simulink model "Simul_BASE_XLS_animation"  (R2016b)
settings: Solver=FixedStepAuto  StartTime=0.0  StopTime=60  FixedStep=0.1  RelTol=1e-3  EnableMultiTasking=on
values from neighbouring files (symbols this model uses):
  attitude_0 = [0,0,0]    [ga_detumbling.m]    (also in ga_detumbling_fit.m = [0.0524,-0.0349,0.0175]; ga_pid.m; ga_pid_fit.m; ga_pid_test.m)
  attitude_rate_0 = [0,6.7e-05,0.0041]    [ga_detumbling.m]    (also in ga_detumbling_fit.m = [0.0873,-0.0873,-0.0873]; ga_pid.m; ga_pid_fit.m; ga_pid_test.m)
  dp = x(2)    [ga_detumbling.m]    (also in ga_detumbling_fit.m = d(2); ga_pid.m = x(4); ga_pid_fit.m = d(4); ga_pid_test.m = x(4))
  dr = x(1)    [ga_detumbling.m]    (also in ga_detumbling_fit.m = d(1); ga_pid.m = x(2); ga_pid_fit.m = d(2); ga_pid_test.m = x(2))
  dy = x(3)    [ga_detumbling.m]    (also in ga_detumbling_fit.m = d(3); ga_pid.m = x(6); ga_pid_fit.m = d(6); ga_pid_test.m = x(6))
  override = 2    [ga_pid_fit.m]    (also in ga_pid_test.m; init_var.m)
  pp = x(3)    [ga_pid.m]    (also in ga_pid_fit.m = d(3); ga_pid_test.m; init_var.m = 0.6885)
  pr = x(1)    [ga_pid.m]    (also in ga_pid_fit.m = d(1); ga_pid_test.m; init_var.m = 0.8646)
  py = x(5)    [ga_pid.m]    (also in ga_pid_fit.m = d(5); ga_pid_test.m; init_var.m = 0.371)
  slew = [60 0 0]    [ga_detumbling.m]    (also in ga_pid.m; ga_pid_fit.m; ga_pid_test.m)
libraries: simulink_extras x10, aerolibanim x1, simulink x1, aerolibutil x1
CloseFcn:
  | rtwprivate ssgencode ModelCloseRequest Simul_BASE_3MW
settings Model: Creator=Kendrick  LastModifiedBy=ehernandez
settings SolverCC: MaxConsecutiveMinStep=5  ZeroCrossAlgorithm=Adaptive
settings DataIOCC: LimitDataPoints=on  SaveFormat=Array  SignalLoggingSaveFormat=ModelDataLogs
settings OptimizationCC: ExpressionDepthLimit=2147483647  LifeSpan=inf
settings DebuggingCC: AlgebraicLoopMsg=none  UnderspecifiedInitializationDetection=Classic  MergeDetectMultiDrivingBlocksExec=none  SolverPrmCheckMsg=warning  FcnCallInpInsideContextMsg=warning  StateNameClashWarn=warning  SFUnexpectedBacktrackingDiag=warning  SFNoUnconditionalDefaultTransitionDiag=warning  SFExecutionAtInitializationDiag=none
settings HardwareCC: ProdBitPerInt=16  ProdBitPerPointer=16  ProdBitPerSizeT=16  ProdBitPerPtrDiffT=16  ProdLargestAtomicFloat=None  ProdIntDivRoundTo=Undefined  ProdEndianess=Unspecified  ProdWordSize=16  ProdHWDeviceType=Generic->16-bit Embedded Processor
settings ModelReferenceCC: PropagateSignalLabelsOutOfModel=off
settings GRTTargetCC: TargetLangStandard=C89/C90 (ANSI)  GeneratePreprocessorConditionals=Disable all  CombineOutputUpdateFcns=off  GRTInterface=on
settings ConfigComp: CovMetricSettings=dw  CovHtmlReporting=on  CovSaveCumulativeToWorkspaceVar=on  CovSaveSingleToWorkspaceVar=on  CovExternalEMLEnable=off
settings SimscapeCC: ExplicitSolverDiagnosticOptions=error  GlobalZcOffDiagnosticOptions=error
settings SimMechanicsCC: VisOnUpdateDiagram=on  VisDuringSimulation=on  LastVizWinPosition=[824 49 610 743]  CamPosition=[0.0449883;0.218364;11.4685;]  CamTarget=[-0.000193585;-0.0218554;-0.00055518;]  CamUpVector=[-0.0100593;0.999731;-0.0208998;]  CamHeight=0.706401  VisBackgroundColor=[0.9;0.9;0.95;]  DefaultBodyColor=[1;0;0;]
settings ConfigurationSet: Description=SimMechanics 2G

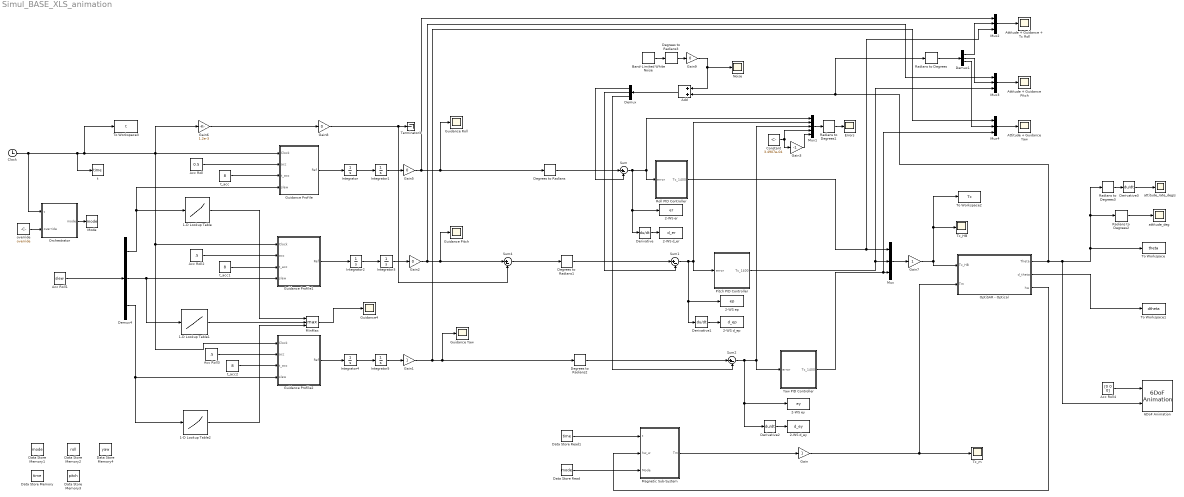
== system Simul_BASE_XLS_animation ==
  1-D Lookup Table : Lookup_n-D  NumberOfTableDimensions=1  BreakpointsForDimension1=[0,10,20,30,60,90]  Table=[0,18,22,25,30,34]  InterpMethod=Cubic spline  ExtrapMethod=Cubic spline  InternalRulePriority=Speed  RndMeth=Simplest  InputSameDT=on
  1-D Lookup Table1 : Lookup_n-D  NumberOfTableDimensions=1  BreakpointsForDimension1=[0,30,60,90]  Table=[0,25,30,34]  InterpMethod=Cubic spline  ExtrapMethod=Cubic spline  InternalRulePriority=Speed  RndMeth=Simplest  InputSameDT=on
  1-D Lookup Table2 : Lookup_n-D  NumberOfTableDimensions=1  BreakpointsForDimension1=[0,30,60,90]  Table=[0,25,30,34]  InterpMethod=Cubic spline  ExtrapMethod=Cubic spline  InternalRulePriority=Speed  RndMeth=Simplest  InputSameDT=on
  2-WS d_ep : ToWorkspace  VariableName=d_ep  SampleTime=-1
  2-WS d_er : ToWorkspace  VariableName=d_er  SampleTime=-1
  2-WS d_ey : ToWorkspace  VariableName=d_ey  SampleTime=-1
  2-WS ep : ToWorkspace  VariableName=ep  SampleTime=-1
  2-WS er : ToWorkspace  VariableName=er  SampleTime=-1
  2-WS ey : ToWorkspace  VariableName=ey  SampleTime=-1
  6DoF Animation : aerolibanim/6DoF Animation  u1=[0 40 -20 20 -50 -30]  u2=0.1  u3=10  u4=[40 0.00 -50]  u5=Fixed position  u6=[20 5 -31.5]  u7=10  u8=on
  Acc Roll : Constant  Value=0.5
  Acc Roll1 : Constant  Value=slew  VectorParams1D=off
  Acc Roll2 : Constant  Value=.5
  Acc Roll3 : Constant  Value=.5
  Acc Roll4 : Constant  Value=[0 0 0]
  Add : Sum
  Attitude + Guidance Pitch : Scope
  Attitude + Guidance Yaw : Scope
  Attitude + Guidance + Tc Roll : Scope
  Band-Limited White Noise : simulink/Sources/Band-Limited White Noise  Cov=[6.4e-4]  Ts=0.1  seed=[23341]  VectorParams1D=off
  Clock : Clock
  Constant : Constant  Value=3.4907e-04
  Data Store Memory : DataStoreMemory  DataStoreName=time  ReadBeforeWriteMsg=warning  WriteAfterWriteMsg=warning  WriteAfterReadMsg=warning  ShowAdditionalParam=off
  Data Store Memory1 : DataStoreMemory  DataStoreName=mode  ReadBeforeWriteMsg=warning  WriteAfterWriteMsg=warning  WriteAfterReadMsg=warning  ShowAdditionalParam=off
  Data Store Memory2 : DataStoreMemory  DataStoreName=roll  ReadBeforeWriteMsg=warning  WriteAfterWriteMsg=warning  WriteAfterReadMsg=warning  ShowAdditionalParam=off
  Data Store Memory3 : DataStoreMemory  DataStoreName=pitch  ReadBeforeWriteMsg=warning  WriteAfterWriteMsg=warning  WriteAfterReadMsg=warning  ShowAdditionalParam=off
  Data Store Memory4 : DataStoreMemory  DataStoreName=yaw  ReadBeforeWriteMsg=warning  WriteAfterWriteMsg=warning  WriteAfterReadMsg=warning  ShowAdditionalParam=off
  Data Store Read : DataStoreRead  DataStoreName=mode
  Data Store Read1 : DataStoreRead  DataStoreName=time  DataStoreElements=time
  Degrees to Radians{,1..3} (4 alike) : simulink_extras/Transformations/Degrees to Radians
  Demux : Demux  Outputs=3
  Demux1 : Demux  Outputs=3
  Demux4 : Demux  Outputs=3
  Derivative{,1..3} (4 alike) : Derivative
  Errors : Scope
  Gain : Gain
  Gain1 : Gain
  Gain{2,5,8..9} (4 alike) : Gain  Gain=0
  Gain3 : Gain  Gain=-1
  Gain6 : Gain  Gain=1.2e-3
  Gain7 : Gain
  Guidance Pitch : Scope
  Guidance Profile : MATLAB Function  TreatAsAtomicUnit=on
  Guidance Profile1 : MATLAB Function  TreatAsAtomicUnit=on
  Guidance Profile2 : MATLAB Function  TreatAsAtomicUnit=on
  Guidance Roll : Scope
  Guidance Yaw : Scope
  Guidance4 : Scope
  Integrator{,1..5} (6 alike) : Integrator
  Magnetic Sub-System : Subsystem
  MinMax : MinMax  Function=max  Inputs=3
  Mode : DataStoreWrite  DataStoreName=mode
  Mux{,2..4} (4 alike) : Mux  Inputs=3
  Mux1 : Mux  Inputs=5
  Noise : Scope
  OptiSAR - Optical : Subsystem
  Orchestrator : MATLAB Function  TreatAsAtomicUnit=on
  Pitch PID Controller : Subsystem
  Radians to Degrees{,1..3} (4 alike) : simulink_extras/Transformations/Radians to Degrees
  Roll PID Controller : Subsystem
  Sum{,1..2,4} (4 alike) : Sum  Inputs=|+-
  Tc_HB : Scope
  Tc_m : Scope
  Terminator3 : Terminator
  To Workspace : ToWorkspace  VariableName=theta  SampleTime=-1
  To Workspace1 : ToWorkspace  VariableName=dtheta  SampleTime=-1
  To Workspace2 : ToWorkspace  VariableName=Tc  SampleTime=-1
  To Workspace3 : ToWorkspace  VariableName=t  SampleTime=-1
  Yaw PID Controller : Subsystem
  attitude_deg : Scope
  attitude_rate_deg/s : Scope
  override : Constant  Value=override  VectorParams1D=off
  t : DataStoreWrite  DataStoreName=time  DataStoreElements=time
  t_acc : Constant  Value=8
  t_acc1 : Constant  Value=8
  t_acc2 : Constant  Value=8
  wires:
  Sum/1 -> Mux1/1, Roll PID Controller/1(error), Derivative/1, 2-WS er/1
  Sum2/1 -> Yaw PID Controller/1(error), Mux1/3, Derivative2/1, 2-WS ey/1
  Demux/3 -> Sum2/2
  OptiSAR - Optical/1(Theta) -> Radians to Degrees/1, Add/2, 6DoF Animation/2, To Workspace/1, Radians to Degrees2/1, Radians to Degrees3/1
  Degrees to Radians2/1 -> Sum2/1
  Demux/1 -> Sum/2
  Derivative/1 -> 2-WS d_er/1
  Derivative1/1 -> 2-WS d_ep/1
  Derivative2/1 -> 2-WS d_ey/1
  Pitch PID Controller/1(Tc_1400) -> Mux3/3, Mux/2
  OptiSAR - Optical/2(d_theta) -> To Workspace1/1
  Guidance Profile/1(Ref) -> Integrator/1
  Integrator3/1 -> Gain2/1
  Mux1/1 -> Radians to Degrees1/1
  Radians to Degrees1/1 -> Errors/1
  Mux2/1 -> Attitude + Guidance + Tc Roll/1
  Integrator5/1 -> Gain1/1
  Integrator/1 -> Integrator1/1
  Integrator1/1 -> Gain5/1
  Guidance Profile1/1(Ref) -> Integrator2/1
  Integrator2/1 -> Integrator3/1
  Guidance Profile2/1(Ref) -> Integrator4/1
  Integrator4/1 -> Integrator5/1
  Radians to Degrees/1 -> Demux1/1
  Demux1/1 -> Mux2/2
  Mux3/1 -> Attitude + Guidance Pitch/1
  Mux4/1 -> Attitude + Guidance Yaw/1
  Demux1/3 -> Mux4/2
  Demux1/2 -> Mux3/2
  Mux/1 -> Gain7/1
  Constant/1 -> Gain3/1, Mux1/4
  Gain3/1 -> Mux1/5
  Sum1/1 -> Derivative1/1, 2-WS ep/1, Pitch PID Controller/1(error), Mux1/2
  Roll PID Controller/1(Tc_1400) -> Mux2/3, Mux/1
  Clock/1 -> Orchestrator/1(t), t/1, Guidance Profile/1(Clock), Gain6/1, Guidance Profile1/1(Clock), Guidance Profile2/1(Clock), To Workspace3/1
  Acc Roll/1 -> Guidance Profile/2(acc)
  Acc Roll2/1 -> Guidance Profile1/2(acc)
  Acc Roll3/1 -> Guidance Profile2/2(acc)
  Acc Roll1/1 -> Demux4/1
  Demux4/1 -> 1-D Lookup Table/1, Guidance Profile/4(slew)
  Demux4/2 -> 1-D Lookup Table1/1, Guidance Profile1/4(slew)
  Demux4/3 -> 1-D Lookup Table2/1, Guidance Profile2/4(slew)
  Gain1/1 -> Guidance Yaw/1, Degrees to Radians2/1, Mux4/1
  t_acc/1 -> Guidance Profile/3(t_acc)
  Gain2/1 -> Mux3/1, Sum4/1, Guidance Pitch/1
  t_acc1/1 -> Guidance Profile1/3(t_acc)
  t_acc2/1 -> Guidance Profile2/3(t_acc)
  Gain5/1 -> Mux2/1, Degrees to Radians/1, Guidance Roll/1
  MinMax/1 -> Guidance4/1
  1-D Lookup Table/1 -> MinMax/1
  1-D Lookup Table1/1 -> MinMax/2
  1-D Lookup Table2/1 -> MinMax/3
  Degrees to Radians/1 -> Sum/1
  Degrees to Radians1/1 -> Sum1/1
  Demux/2 -> Sum1/2
  OptiSAR - Optical/3(hw) -> Magnetic Sub-System/2(hw_w)
  Gain/1 -> Tc_m/1, OptiSAR - Optical/2(Tm)
  Gain6/1 -> Gain8/1
  Sum4/1 -> Degrees to Radians1/1
  Gain7/1 -> OptiSAR - Optical/1(Tc_HB), To Workspace2/1, Tc_HB/1
  Gain8/1 -> Sum4/2, Terminator3/1
  Derivative3/1 -> attitude_rate_deg/s/1
  Radians to Degrees2/1 -> attitude_deg/1
  Radians to Degrees3/1 -> Derivative3/1
  Magnetic Sub-System/1(Tm) -> Gain/1
  Yaw PID Controller/1(Tc_1400) -> Mux4/3, Mux/3
  Data Store Read1/1 -> Magnetic Sub-System/1(t)
  Orchestrator/1(mode) -> Mode/1
  override/1 -> Orchestrator/2(override)
  Data Store Read/1 -> Magnetic Sub-System/3(Mode)
  Acc Roll4/1 -> 6DoF Animation/1
  Band-Limited White Noise/1 -> Degrees to Radians3/1
  Add/1 -> Demux/1
  Degrees to Radians3/1 -> Gain9/1
  Gain9/1 -> Add/1, Noise/1

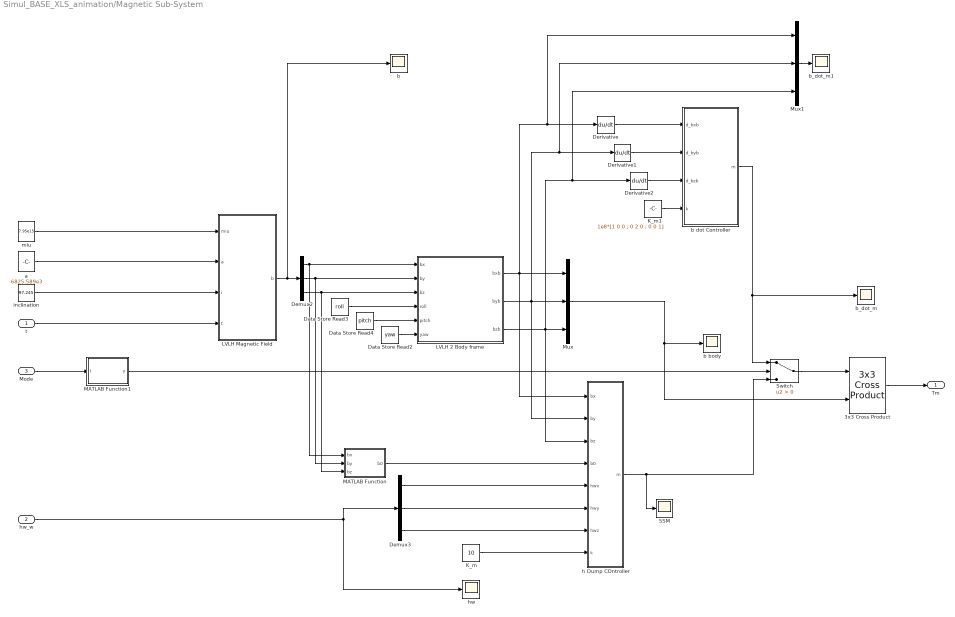
== system Simul_BASE_XLS_animation/Magnetic Sub-System ==
  t : Inport
  hw_w : Inport  Port=2
  Mode : Inport  Port=3
  3x3 Cross Product : aerolibutil/3x3 Cross Product
  Data Store Read2 : DataStoreRead  DataStoreName=yaw
  Data Store Read3 : DataStoreRead  DataStoreName=roll
  Data Store Read4 : DataStoreRead  DataStoreName=pitch
  Demux2 : Demux  Outputs=3
  Demux3 : Demux  Outputs=3
  Derivative : Derivative
  Derivative1 : Derivative
  Derivative2 : Derivative
  K_m : Constant  Value=10
  K_m1 : Constant  Value=1e8*[1 0 0 ; 0 2 0 ; 0 0 1]
  LVLH 2 Body frame : MATLAB Function  TreatAsAtomicUnit=on
  LVLH Magnetic Field : MATLAB Function  TreatAsAtomicUnit=on
  MATLAB Function : MATLAB Function  TreatAsAtomicUnit=on
  MATLAB Function1 : MATLAB Function  TreatAsAtomicUnit=on
  Mux : Mux  Inputs=3
  Mux1 : Mux  Inputs=3
  SSM : Scope
  Switch : Switch  Criteria=u2 > Threshold
  a : Constant  Value=6825.589e3
  b : Scope
  b body : Scope
  b dot Controller : MATLAB Function  TreatAsAtomicUnit=on
  b_dot_m : Scope
  b_dot_m1 : Scope
  h Dump COntroller : MATLAB Function  TreatAsAtomicUnit=on
  hw : Scope
  inclination : Constant  Value=97.245
  miu : Constant  Value=7.95e15
  Tm : Outport
  wires:
  Demux3/3 -> h Dump COntroller/7(hwz)
  hw_w/1 -> hw/1, Demux3/1
  Demux3/2 -> h Dump COntroller/6(hwy)
  inclination/1 -> LVLH Magnetic Field/3(i)
  t/1 -> LVLH Magnetic Field/4(t)
  Demux2/1 -> MATLAB Function/1(bx), LVLH 2 Body frame/1(bx)
  Demux2/2 -> MATLAB Function/2(by), LVLH 2 Body frame/2(by)
  Demux2/3 -> MATLAB Function/3(bz), LVLH 2 Body frame/3(bz)
  LVLH Magnetic Field/1(b) -> Demux2/1, b/1
  miu/1 -> LVLH Magnetic Field/1(miu)
  K_m/1 -> h Dump COntroller/8(k)
  Demux3/1 -> h Dump COntroller/5(hwx)
  a/1 -> LVLH Magnetic Field/2(a)
  MATLAB Function/1(b0) -> h Dump COntroller/4(b0)
  K_m1/1 -> b dot Controller/4(k)
  Mode/1 -> MATLAB Function1/1(t)
  Derivative/1 -> b dot Controller/1(d_bxb)
  Derivative1/1 -> b dot Controller/2(d_byb)
  Derivative2/1 -> b dot Controller/3(d_bzb)
  Switch/1 -> 3x3 Cross Product/1
  Mux/1 -> b body/1, 3x3 Cross Product/2
  h Dump COntroller/1(m) -> SSM/1, Switch/3
  b dot Controller/1(m) -> Switch/1, b_dot_m/1
  3x3 Cross Product/1 -> Tm/1
  MATLAB Function1/1(y) -> Switch/2
  Data Store Read3/1 -> LVLH 2 Body frame/4(roll)
  Data Store Read4/1 -> LVLH 2 Body frame/5(pitch)
  Data Store Read2/1 -> LVLH 2 Body frame/6(yaw)
  LVLH 2 Body frame/1(bxb) -> h Dump COntroller/1(bx), Mux1/1, Derivative/1, Mux/1
  LVLH 2 Body frame/2(byb) -> h Dump COntroller/2(by), Mux1/2, Derivative1/1, Mux/2
  LVLH 2 Body frame/3(bzb) -> h Dump COntroller/3(bz), Mux1/3, Derivative2/1, Mux/3
  Mux1/1 -> b_dot_m1/1

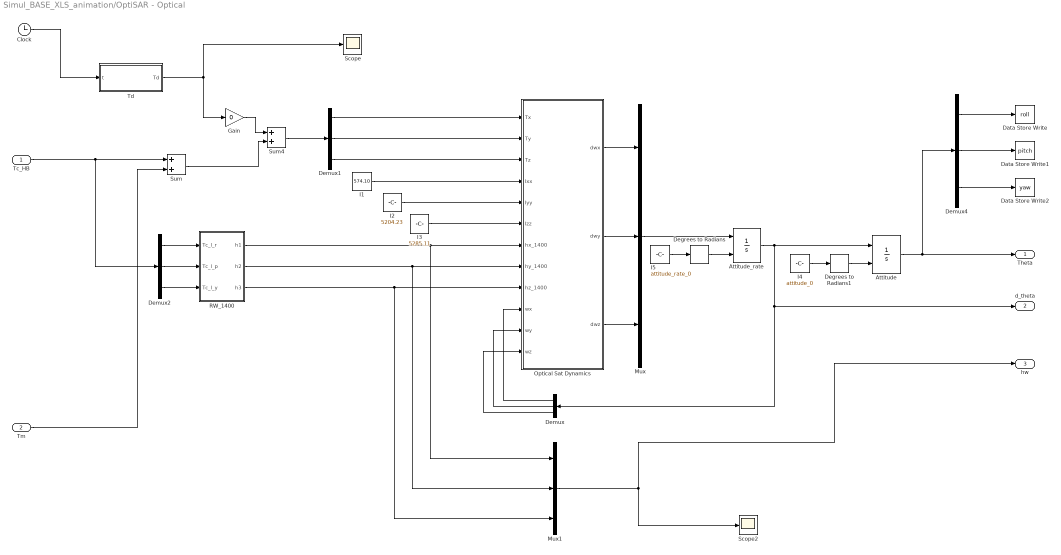
== system Simul_BASE_XLS_animation/OptiSAR - Optical ==
  Tc_HB : Inport
  Tm : Inport  Port=2
  Attitude : Integrator  InitialConditionSource=external
  Attitude_rate : Integrator  InitialConditionSource=external
  Clock : Clock
  Data Store Write : DataStoreWrite  DataStoreName=roll
  Data Store Write1 : DataStoreWrite  DataStoreName=pitch
  Data Store Write2 : DataStoreWrite  DataStoreName=yaw
  Degrees to Radians : simulink_extras/Transformations/Degrees to Radians
  Degrees to Radians1 : simulink_extras/Transformations/Degrees to Radians
  Demux{,1..2,4} (4 alike) : Demux  Outputs=3
  Gain : Gain  Gain=0
  I1 : Constant  Value=574.10
  I2 : Constant  Value=5204.23
  I3 : Constant  Value=5285.11
  I4 : Constant  Value=attitude_0
  I5 : Constant  Value=attitude_rate_0
  Mux : Mux  Inputs=3
  Mux1 : Mux  Inputs=3
  Optical Sat Dynamics : MATLAB Function  TreatAsAtomicUnit=on
  RW_1400 : Subsystem
  Scope : Scope
  Scope2 : Scope
  Sum : Sum
  Sum4 : Sum
  Td : Subsystem
  Theta : Outport
  d_theta : Outport  Port=2
  hw : Outport  Port=3
  wires:
  Clock/1 -> Td/1(t)
  Attitude/1 -> Demux4/1, Theta/1
  Attitude_rate/1 -> Demux/1, d_theta/1, Attitude/1
  I3/1 -> Optical Sat Dynamics/6(Izz)
  I2/1 -> Optical Sat Dynamics/5(Iyy)
  I1/1 -> Optical Sat Dynamics/4(Ixx)
  Demux/1 -> Optical Sat Dynamics/10(wx)
  Demux/2 -> Optical Sat Dynamics/11(wy)
  Demux/3 -> Optical Sat Dynamics/12(wz)
  Optical Sat Dynamics/1(dwx) -> Mux/1
  Optical Sat Dynamics/2(dwy) -> Mux/2
  Optical Sat Dynamics/3(dwz) -> Mux/3
  Mux/1 -> Attitude_rate/1
  Td/1(Td) -> Gain/1, Scope/1
  Demux1/1 -> Optical Sat Dynamics/1(Tx)
  Demux1/2 -> Optical Sat Dynamics/2(Ty)
  Demux1/3 -> Optical Sat Dynamics/3(Tz)
  Demux2/1 -> RW_1400/1(Tc_l_r)
  Demux2/2 -> RW_1400/2(Tc_l_p)
  Demux2/3 -> RW_1400/3(Tc_l_y)
  Sum/1 -> Sum4/2
  Tm/1 -> Sum/2
  Mux1/1 -> hw/1, Scope2/1
  Tc_HB/1 -> Demux2/1, Sum/1
  I4/1 -> Degrees to Radians1/1
  RW_1400/1(h1) -> Mux1/1, Optical Sat Dynamics/7(hx_1400)
  RW_1400/3(h3) -> Mux1/3, Optical Sat Dynamics/9(hz_1400)
  RW_1400/2(h2) -> Mux1/2, Optical Sat Dynamics/8(hy_1400)
  I5/1 -> Degrees to Radians/1
  Degrees to Radians/1 -> Attitude_rate/2
  Degrees to Radians1/1 -> Attitude/2
  Sum4/1 -> Demux1/1
  Gain/1 -> Sum4/1
  Demux4/1 -> Data Store Write/1
  Demux4/2 -> Data Store Write1/1
  Demux4/3 -> Data Store Write2/1

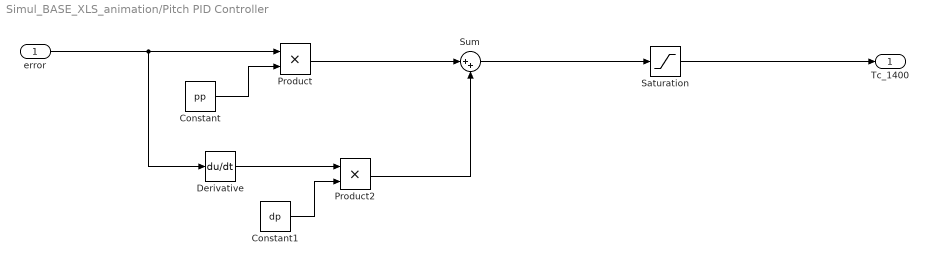
== system Simul_BASE_XLS_animation/Pitch PID Controller ==
  error : Inport
  Constant : Constant  Value=pp
  Constant1 : Constant  Value=dp
  Derivative : Derivative
  Product : Product
  Product2 : Product
  Saturation : Saturate  UpperLimit=5.21  LowerLimit=-5.21
  Sum : Sum  Inputs=|++
  Tc_1400 : Outport
  wires:
  Sum/1 -> Saturation/1
  Product2/1 -> Sum/2
  Product/1 -> Sum/1
  Constant/1 -> Product/2
  Constant1/1 -> Product2/2
  Derivative/1 -> Product2/1
  error/1 -> Derivative/1, Product/1
  Saturation/1 -> Tc_1400/1

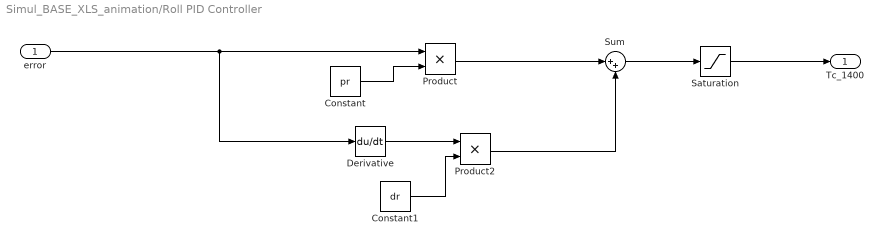
== system Simul_BASE_XLS_animation/Roll PID Controller ==
  error : Inport
  Constant : Constant  Value=pr
  Constant1 : Constant  Value=dr
  Derivative : Derivative
  Product : Product
  Product2 : Product
  Saturation : Saturate  UpperLimit=3.23  LowerLimit=-3.23
  Sum : Sum  Inputs=|++
  Tc_1400 : Outport
  wires:
  Sum/1 -> Saturation/1
  Product2/1 -> Sum/2
  Product/1 -> Sum/1
  Constant/1 -> Product/2
  Constant1/1 -> Product2/2
  Derivative/1 -> Product2/1
  Saturation/1 -> Tc_1400/1
  error/1 -> Derivative/1, Product/1

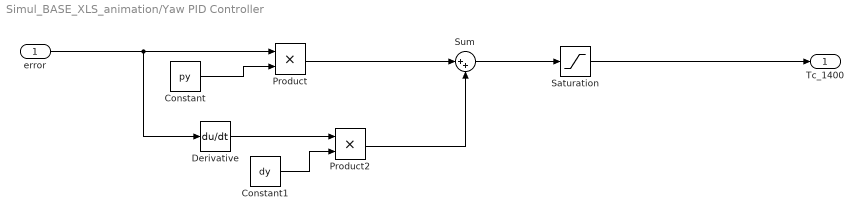
== system Simul_BASE_XLS_animation/Yaw PID Controller ==
  error : Inport
  Constant : Constant  Value=py
  Constant1 : Constant  Value=dy
  Derivative : Derivative
  Product : Product
  Product2 : Product
  Saturation : Saturate  UpperLimit=5.21  LowerLimit=-5.21
  Sum : Sum  Inputs=|++
  Tc_1400 : Outport
  wires:
  Sum/1 -> Saturation/1
  Product2/1 -> Sum/2
  Product/1 -> Sum/1
  Constant/1 -> Product/2
  Constant1/1 -> Product2/2
  Derivative/1 -> Product2/1
  error/1 -> Product/1, Derivative/1
  Saturation/1 -> Tc_1400/1

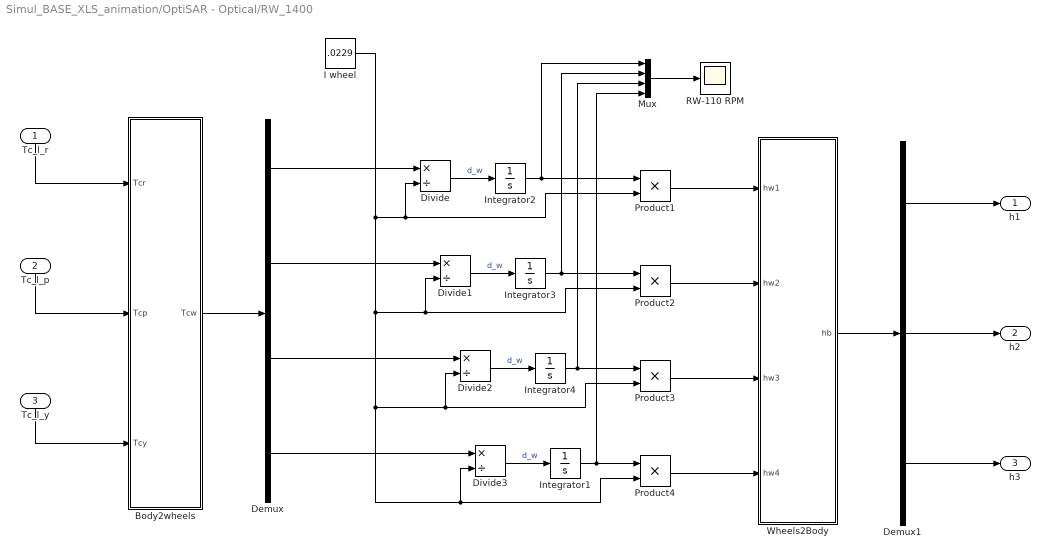
== system Simul_BASE_XLS_animation/OptiSAR - Optical/RW_1400 ==
  Tc_l_r : Inport
  Tc_l_p : Inport  Port=2
  Tc_l_y : Inport  Port=3
  Body2wheels : MATLAB Function  TreatAsAtomicUnit=on
  Demux : Demux
  Demux1 : Demux  Outputs=3
  Divide{,1..3} (4 alike) : Product  Inputs=*/
  I wheel : Constant  Value=.0229
  Integrator{1..4} (4 alike) : Integrator
  Mux : Mux
  Product{1..4} (4 alike) : Product
  RW-110 RPM : Scope
  Wheels2Body : MATLAB Function  TreatAsAtomicUnit=on
  h1 : Outport
  h2 : Outport  Port=2
  h3 : Outport  Port=3
  wires:
  Divide2/1 -> Integrator4/1  "d_w"
  Integrator4/1 -> Product3/1, Mux/3
  Integrator3/1 -> Mux/2, Product2/1
  Divide1/1 -> Integrator3/1  "d_w"
  Integrator2/1 -> Mux/1, Product1/1
  Divide/1 -> Integrator2/1  "d_w"
  Tc_l_p/1 -> Body2wheels/2(Tcp)
  Tc_l_r/1 -> Body2wheels/1(Tcr)
  Tc_l_y/1 -> Body2wheels/3(Tcy)
  Divide3/1 -> Integrator1/1  "d_w"
  I wheel/1 -> Divide3/2, Product4/2, Divide2/2, Product3/2, Divide1/2, Product2/2, Divide/2, Product1/2
  Integrator1/1 -> Product4/1, Mux/4
  Body2wheels/1(Tcw) -> Demux/1
  Demux/1 -> Divide/1
  Demux/2 -> Divide1/1
  Demux/3 -> Divide2/1
  Demux/4 -> Divide3/1
  Demux1/1 -> h1/1
  Demux1/2 -> h2/1
  Demux1/3 -> h3/1
  Wheels2Body/1(hb) -> Demux1/1
  Product1/1 -> Wheels2Body/1(hw1)
  Product2/1 -> Wheels2Body/2(hw2)
  Product3/1 -> Wheels2Body/3(hw3)
  Product4/1 -> Wheels2Body/4(hw4)
  Mux/1 -> RW-110 RPM/1

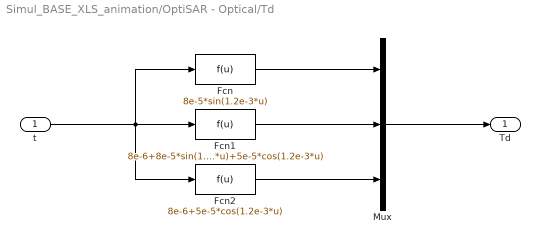
== system Simul_BASE_XLS_animation/OptiSAR - Optical/Td ==
  t : Inport
  Fcn : Fcn  Expr=8e-5*sin(1.2e-3*u)
  Fcn1 : Fcn  Expr=8e-6+8e-5*sin(1.2e-3*u)+5e-5*cos(1.2e-3*u)
  Fcn2 : Fcn  Expr=8e-6+5e-5*cos(1.2e-3*u)
  Mux : Mux  Inputs=3
  Td : Outport
  wires:
  t/1 -> Fcn1/1, Fcn/1, Fcn2/1
  Fcn1/1 -> Mux/2
  Fcn/1 -> Mux/1
  Fcn2/1 -> Mux/3
  Mux/1 -> Td/1

== matlab function Simul_BASE_XLS_animation/OptiSAR - Optical/Optical Sat Dynamics ==
  data: Tx input; Ty input; Tz input; Ixx input; Iyy input; Izz input; hx_1400 input; hy_1400 input; hz_1400 input; wx input; wy input; wz input; dwx output; dwy output; dwz output
function [dwx,dwy,dwz] = Satellite(Tx,Ty,Tz,Ixx,Iyy,Izz,hx_1400,hy_1400,hz_1400,wx,wy,wz)

dwx = (Tx-(Iyy-Izz)*wz*wy+(hz_1400)*wy-(hy_1400)*wz)/Ixx;
dwy = (Ty-(Izz-Ixx)*wx*wz+(hx_1400)*wz-(hz_1400)*wx)/Iyy;
dwz = (Tz-(Ixx-Iyy)*wy*wx+(hy_1400)*wx-(hx_1400)*wy)/Izz;

== matlab function Simul_BASE_XLS_animation/Guidance Profile ==
  data: Clock input; Ref output; acc input; t_acc input; slew input
function Ref = Guidance(Clock,acc,t_acc,slew)
u=0;
t_c=(slew/acc-t_acc^2)/t_acc;

if Clock<t_acc
    u=acc;
end

if Clock>=t_acc+t_c&&Clock<2*t_acc+t_c
    u=-acc;
end
if slew==0
    Ref = 0;
else
    Ref = u;
end

== matlab function Simul_BASE_XLS_animation/Guidance Profile1 ==
  data: Clock input; Ref output; acc input; t_acc input; slew input
function Ref = Guidance(Clock,acc,t_acc,slew)
u=0;
t_c=(slew/acc-t_acc^2)/t_acc;

if Clock<t_acc
    u=acc;
end

if Clock>=t_acc+t_c&&Clock<2*t_acc+t_c
    u=-acc;
end
if slew==0
    Ref = 0;
else
    Ref = u;
end

== matlab function Simul_BASE_XLS_animation/Guidance Profile2 ==
  data: Clock input; Ref output; acc input; t_acc input; slew input
function Ref = Guidance(Clock,acc,t_acc,slew)
u=0;
t_c=(slew/acc-t_acc^2)/t_acc;

if Clock<t_acc
    u=acc;
end

if Clock>=t_acc+t_c&&Clock<2*t_acc+t_c
    u=-acc;
end

if slew==0
    Ref = 0;
else
    Ref = u;
end

== matlab function Simul_BASE_XLS_animation/Magnetic Sub-System/LVLH 2 Body frame ==
  data: bx input; bxb output; by input; bz input; roll input; pitch input; yaw input; byb output; bzb output
function [bxb,byb,bzb] = fcn(bx,by,bz,roll,pitch,yaw)
bb=[cos(pitch)          ,-cos(yaw)*sin(pitch)                               ,sin(pitch)*sin(yaw);
    cos(roll)*sin(pitch), cos(roll)*cos(pitch)*cos(yaw)-sin(roll)*sin(yaw)  ,-cos(yaw)*sin(roll)-cos(roll)*cos(pitch)*sin(yaw);
    sin(roll)*sin(pitch), cos(roll)*sin(yaw)+cos(pitch)*cos(yaw)*sin(roll)   , cos(roll)*cos(yaw)-cos(pitch)*sin(roll)*sin(yaw)]*[bx;by;bz];
bxb=bb(1);
byb=bb(2);
bzb=bb(3);

== matlab function Simul_BASE_XLS_animation/Magnetic Sub-System/h Dump COntroller ==
  data: bx input; by input; bz input; b0 input; hwx input; hwy input; hwz input; k input; m output
function m  = fcn(bx,by,bz,b0,hwx, hwy, hwz,k)
m=-k/b0^2*cross([bx ; by ; bz] ,[hwx;hwy;hwz]);
for i=1:3
    if m(i)>110||m(i)<-100
        m(i)=110;
    end
end
%cross(m,[bxb ; byb ; bzb]);

== matlab function Simul_BASE_XLS_animation/OptiSAR - Optical/RW_1400/Body2wheels ==
  data: Tcr input; Tcw output; Tcp input; Tcy input
function Tcw = body2wheels(Tcr,Tcp,Tcy)
Tcw=[0.144325, 0.144325, -0.144325;
     0.144325, -0.144325, -0.144325;
     -0.144325, -0.144325, -0.144325;
     -0.144325, 0.144325, -0.144325]*[Tcr;Tcp;Tcy];

== matlab function Simul_BASE_XLS_animation/OptiSAR - Optical/RW_1400/Wheels2Body ==
  data: hw1 input; hb output; hw2 input; hw3 input; hw4 input
function hb = wheels2body(hw1,hw2,hw3,hw4)
hb= [0.5774 , 0.5774 , -0.5774 , -0.5774 ;
     0.5774 , -0.5774 , -0.5774 , 0.5774;
    -0.5774 , -0.5774 , -0.5774 , -0.5774]*[hw1;hw2;hw3;hw4];

== matlab function Simul_BASE_XLS_animation/Magnetic Sub-System/LVLH Magnetic Field ==
  data: miu input; a input; i input; b output; t input
function b = magnetic_field(miu,a,i,t)

b = miu/a^3*[sin(deg2rad(i))*cos(1.2e-3*t);
    -cos(deg2rad(i));
    2*sin(deg2rad(i))*sin(1.2e-3*t)];

== matlab function Simul_BASE_XLS_animation/Magnetic Sub-System/b dot Controller ==
  data: d_bxb input; d_byb input; d_bzb input; k input; m output
function m = fcn(d_bxb, d_byb, d_bzb, k)
m=-k*[d_bxb ;d_byb ;d_bzb];
for i=1:3
    if m(i)>110
        m(i)=110;
    end
    if m(i)<-110
        m(i)=-110;
    end
end
%cross(m,[bxb ; byb ; bzb]);

== matlab function Simul_BASE_XLS_animation/Magnetic Sub-System/MATLAB Function1 ==
  data: t input; y output
function y = fcn(t)
y=1;
if t>=10000
    y=-1;
end

== matlab function Simul_BASE_XLS_animation/Magnetic Sub-System/MATLAB Function ==
  data: bx input; b0 output; by input; bz input
function b0 = norm(bx,by,bz)

b0 = sqrt(bx^2+by^2+bz^2);

== matlab function Simul_BASE_XLS_animation/Orchestrator ==
  data: t input; mode output; override input
function mode = mode_selector(t,override)
mode=0;
if override~=0
    mode=override;
else    
    if t==0
        mode=0;
    end
    if t>15
        mode=1;
    end
end;
